simulink model "TPS_SWC"  (R2022b)
settings: configuration reference "TPS_AutosarConfig" (kept outside this file)
model workspace (MATLAB code in the model file):
  | cmdLim = Simulink.Parameter;
  | cmdLim.Value = 15;
  | cmdLim.Description = 'Limit for controlling the maximum surface command angle.';
  | cmdLim.Min = 0;
  | cmdLim.Max = 90;
  | cmdLim.DocUnits = 'deg';
  | 
  | dispGain = Simulink.Parameter;
  | dispGain.Value = 0.75;
  | dispGain.Description = 'Gain applied to the displacement error.';
  | dispGain.Min = 0;
  | dispGain.Max = [];
  | dispGain.DocUnits = 'deg/sec/deg';
  | 
  | dispLim = Simulink.Parameter;
  | dispLim.Value = 30;
  | dispLim.Description = 'Limit for controlling the maximum commanded angle.';
  | dispLim.Min = 0;
  | dispLim.Max = 180;
  | dispLim.DocUnits = 'deg';
  | 
  | intGain = Simulink.Parameter;
  | intGain.Value = 0.5;
  | intGain.Description = 'Gain applied to the integral error.';
  | intGain.Min = 0;
  | intGain.Max = [];
  | intGain.DocUnits = 'deg/sec/deg/sec';
  | 
  | intLim = Simulink.Parameter;
  | intLim.Value = 5;
  | intLim.Description = 'Limit for controlling the maximum commanded angle.';
  | intLim.Min = 0;
  | intLim.Max = 90;
  | intLim.DocUnits = 'deg';
  | 
  | rateGain = Simulink.Parameter;
  | rateGain.Value = 2;
  | rateGain.Description = 'Gain applied to the rate error.';
  | rateGain.Min = 0;
  | rateGain.Max = [];
  | rateGain.DocUnits = 'deg/deg/sec';
  | 
  | rateLim = Simulink.Parameter;
  | rateLim.Value = 6;
  | rateLim.Description = 'Limit for controlling the maximum commanded angle.';
  | rateLim.Min = 0;
  | rateLim.Max = 180;
  | rateLim.DocUnits = 'deg/sec';
  | 
  | hdgGain = Simulink.Parameter;
  | hdgGain.Value = 0.015;
values from neighbouring files (symbols this model uses):
  Dem_EventStatusType : value not decoded    [TPS_DD.sldd]
  TPS_SampleTime = 0.01    [TPS_DD.sldd]
libraries: autosarlibdem x4, autosarlibnvm x3, simulink x1
settings Model: RequirementInfo={} %GIDa_fe9045fd_0412_4b6e_8206_617cc20e6fde  DataDictionary=TPS_DD.sldd  FPTRunName=Active  Creator=MAAM  LastModifiedBy=MAAM
settings ConfigSetRef: SourceName=TPS_AutosarConfig

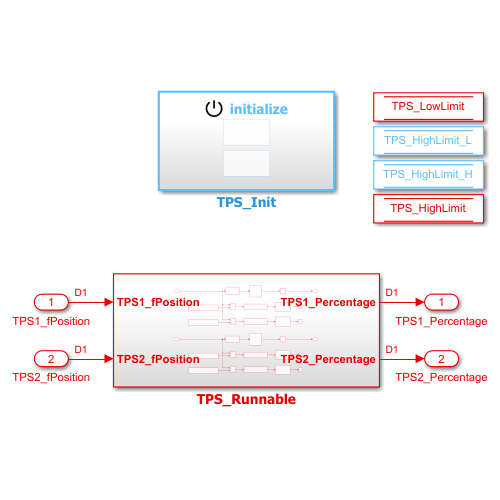
[thumbnail: Simulink's stored preview of the top-level diagram]
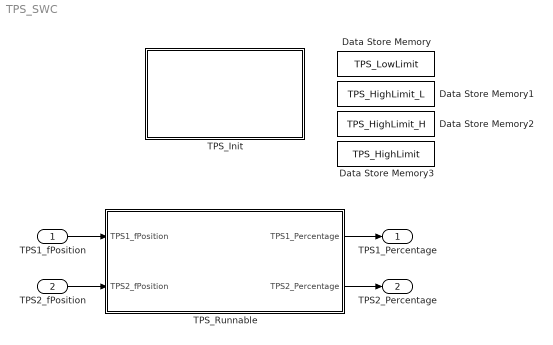
== system TPS_SWC ==
  TPS1_fPosition : Inport  OutDataTypeStr=uint16  SampleTime=TPS_SampleTime
  TPS2_fPosition : Inport  Port=2  OutDataTypeStr=uint16  SampleTime=TPS_SampleTime
  Data Store Memory : DataStoreMemory  DataStoreName=TPS_LowLimit  WriteAfterWriteMsg=warning  ShowAdditionalParam=off  OutDataTypeStr=uint8
  Data Store Memory1 : DataStoreMemory  DataStoreName=TPS_HighLimit_L  WriteAfterWriteMsg=warning  ShowAdditionalParam=off  OutDataTypeStr=uint8
  Data Store Memory2 : DataStoreMemory  DataStoreName=TPS_HighLimit_H  WriteAfterWriteMsg=warning  ShowAdditionalParam=off  OutDataTypeStr=uint8
  Data Store Memory3 : DataStoreMemory  DataStoreName=TPS_HighLimit  WriteAfterWriteMsg=warning  ShowAdditionalParam=off  OutDataTypeStr=uint16
  TPS_Init : Subsystem  TreatAsAtomicUnit=on
  TPS_Runnable : Subsystem  SystemSampleTime=1
  TPS1_Percentage : Outport  OutDataTypeStr=single  Unit=%
  TPS2_Percentage : Outport  Port=2  OutDataTypeStr=single  Unit=%
  wires:
  TPS1_fPosition/1 -> TPS_Runnable/1(TPS1_fPosition)
  TPS2_fPosition/1 -> TPS_Runnable/2(TPS2_fPosition)
  TPS_Runnable/1(TPS1_Percentage) -> TPS1_Percentage/1
  TPS_Runnable/2(TPS2_Percentage) -> TPS2_Percentage/1

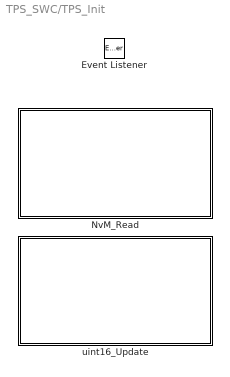
== system TPS_SWC/TPS_Init ==
  Event Listener : EventListener  DisableCoverage=on  EventName=reset
  NvM_Read : Subsystem  Tag=NvM_Read  Priority=1
  uint16_Update : Subsystem  Tag=uint16_Update  Priority=2

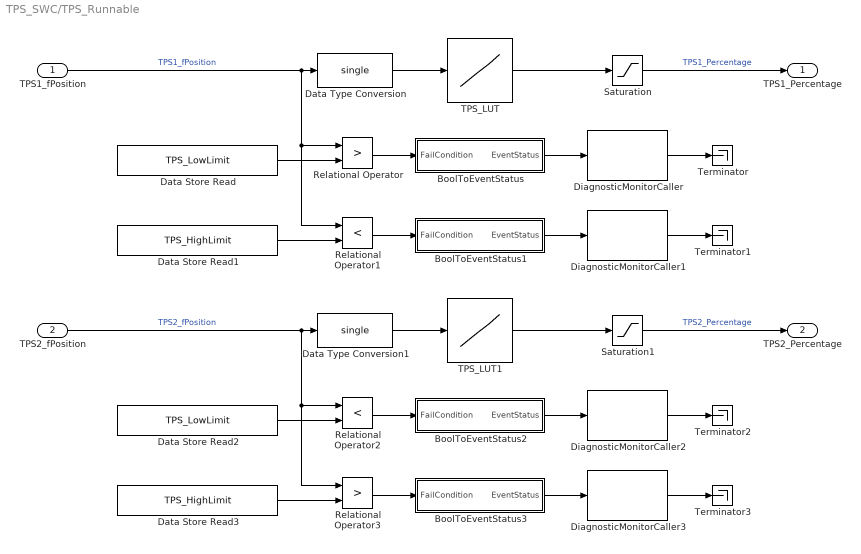
== system TPS_SWC/TPS_Runnable ==
  TPS1_fPosition : Inport  OutDataTypeStr=uint16
  TPS2_fPosition : Inport  Port=2  OutDataTypeStr=uint16
  BoolToEventStatus : Subsystem
  BoolToEventStatus1 : Subsystem
  BoolToEventStatus2 : Subsystem
  BoolToEventStatus3 : Subsystem
  Data Store Read : DataStoreRead  DataStoreName=TPS_LowLimit  IndexOptions=Index vector (dialog)  Indices=1  OutputSizes=1
  Data Store Read1 : DataStoreRead  DataStoreName=TPS_HighLimit  IndexOptions=Index vector (dialog)  Indices=1  OutputSizes=1
  Data Store Read2 : DataStoreRead  DataStoreName=TPS_LowLimit  IndexOptions=Index vector (dialog)  Indices=1  OutputSizes=1
  Data Store Read3 : DataStoreRead  DataStoreName=TPS_HighLimit  IndexOptions=Index vector (dialog)  Indices=1  OutputSizes=1
  Data Type Conversion : DataTypeConversion  OutDataTypeStr=single  SaturateOnIntegerOverflow=off  RndMeth=Floor
  Data Type Conversion1 : DataTypeConversion  OutDataTypeStr=single  SaturateOnIntegerOverflow=off  RndMeth=Floor
  DiagnosticMonitorCaller : autosarlibdem/DiagnosticMonitorCaller  PortName=TPS1_StuckLow  Operation=SetEventStatus  Datatype=Enum: Dem_EventStatusType  st=-1  ServiceImpl=autosar.bsw.DemDiagnosticMonitor
  DiagnosticMonitorCaller1 : autosarlibdem/DiagnosticMonitorCaller  PortName=TPS1_StuckHigh  Operation=SetEventStatus  Datatype=Enum: Dem_EventStatusType  st=-1  ServiceImpl=autosar.bsw.DemDiagnosticMonitor
  DiagnosticMonitorCaller2 : autosarlibdem/DiagnosticMonitorCaller  PortName=TPS2_StuckLow  Operation=SetEventStatus  Datatype=Enum: Dem_EventStatusType  st=-1  ServiceImpl=autosar.bsw.DemDiagnosticMonitor
  DiagnosticMonitorCaller3 : autosarlibdem/DiagnosticMonitorCaller  PortName=TPS2_StuckHigh  Operation=SetEventStatus  Datatype=Enum: Dem_EventStatusType  st=-1  ServiceImpl=autosar.bsw.DemDiagnosticMonitor
  Relational Operator : RelationalOperator  Operator=>  OutDataTypeStr=boolean  RndMeth=Simplest  InputSameDT=off
  Relational Operator1 : RelationalOperator  Operator=<  OutDataTypeStr=boolean  RndMeth=Simplest  InputSameDT=off
  Relational Operator2 : RelationalOperator  Operator=<  OutDataTypeStr=boolean  RndMeth=Simplest  InputSameDT=off
  Relational Operator3 : RelationalOperator  Operator=>  OutDataTypeStr=boolean  RndMeth=Simplest  InputSameDT=off
  Saturation : Saturate  UpperLimit=100  LowerLimit=0
  Saturation1 : Saturate  UpperLimit=100  LowerLimit=0
  TPS_LUT : Lookup_n-D  NumberOfTableDimensions=1  BreakpointsForDimension1=0:100:1000  BreakpointsForDimension1DataTypeStr=single  Table=0:10:100  TableDataTypeStr=single  InterpMethod=Nearest  ExtrapMethod=Clip  InternalRulePriority=Speed  OutDataTypeStr=single  RndMeth=Simplest
  TPS_LUT1 : Lookup_n-D  NumberOfTableDimensions=1  BreakpointsForDimension1=0:100:1000  BreakpointsForDimension1DataTypeStr=single  Table=0:10:100  TableDataTypeStr=single  InterpMethod=Nearest  InternalRulePriority=Speed  OutDataTypeStr=single  RndMeth=Simplest
  Terminator{,1..3} (4 alike) : Terminator
  TPS1_Percentage : Outport  OutDataTypeStr=single  Unit=%
  TPS2_Percentage : Outport  Port=2  OutDataTypeStr=single  Unit=%
  wires:
  Data Type Conversion1/1 -> TPS_LUT1/1
  TPS_LUT1/1 -> Saturation1/1
  Saturation1/1 -> TPS2_Percentage/1  "TPS2_Percentage"
  Data Store Read2/1 -> Relational Operator2/2
  Data Store Read3/1 -> Relational Operator3/2
  TPS2_fPosition/1 -> Relational Operator2/1, Relational Operator3/1, Data Type Conversion1/1  "TPS2_fPosition"
  Relational Operator2/1 -> BoolToEventStatus2/1(FailCondition)
  Relational Operator3/1 -> BoolToEventStatus3/1(FailCondition)
  BoolToEventStatus2/1(EventStatus) -> DiagnosticMonitorCaller2/1
  BoolToEventStatus3/1(EventStatus) -> DiagnosticMonitorCaller3/1
  BoolToEventStatus1/1(EventStatus) -> DiagnosticMonitorCaller1/1
  Relational Operator1/1 -> BoolToEventStatus1/1(FailCondition)
  Relational Operator/1 -> BoolToEventStatus/1(FailCondition)
  TPS1_fPosition/1 -> Data Type Conversion/1, Relational Operator1/1, Relational Operator/1  "TPS1_fPosition"
  Data Store Read1/1 -> Relational Operator1/2
  Data Store Read/1 -> Relational Operator/2
  Saturation/1 -> TPS1_Percentage/1  "TPS1_Percentage"
  TPS_LUT/1 -> Saturation/1
  Data Type Conversion/1 -> TPS_LUT/1
  BoolToEventStatus/1(EventStatus) -> DiagnosticMonitorCaller/1
  DiagnosticMonitorCaller/1 -> Terminator/1
  DiagnosticMonitorCaller1/1 -> Terminator1/1
  DiagnosticMonitorCaller2/1 -> Terminator2/1
  DiagnosticMonitorCaller3/1 -> Terminator3/1

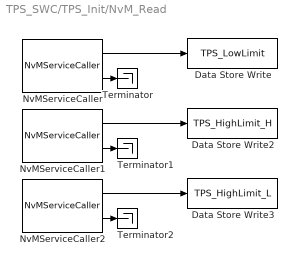
== system TPS_SWC/TPS_Init/NvM_Read ==
  Data Store Write : DataStoreWrite  DataStoreName=TPS_LowLimit  IndexOptions=Index vector (dialog)  Indices=1  OutputSizes=1
  Data Store Write2 : DataStoreWrite  DataStoreName=TPS_HighLimit_H  IndexOptions=Index vector (dialog)  Indices=1  OutputSizes=1
  Data Store Write3 : DataStoreWrite  DataStoreName=TPS_HighLimit_L  IndexOptions=Index vector (dialog)  Indices=1  OutputSizes=1
  NvMServiceCaller : autosarlibnvm/NvMServiceCaller  PortName=TPS_LowLimit_NvMService  Operation=ReadBlock  ArgumentSpecification=TPS_LowLimit_ID  st=-1  ServiceImpl=autosar.bsw.NvMService
  NvMServiceCaller1 : autosarlibnvm/NvMServiceCaller  PortName=TPS_HighLimit_H_NvMService  Operation=ReadBlock  ArgumentSpecification=TPS_HighLimit_ID_H  st=-1  ServiceImpl=autosar.bsw.NvMService
  NvMServiceCaller2 : autosarlibnvm/NvMServiceCaller  PortName=TPS_HighLimit_L_NvMService  Operation=ReadBlock  ArgumentSpecification=TPS_HighLimit_ID_L  st=-1  ServiceImpl=autosar.bsw.NvMService
  Terminator : Terminator
  Terminator1 : Terminator
  Terminator2 : Terminator
  wires:
  NvMServiceCaller1/1 -> Data Store Write2/1
  NvMServiceCaller/2 -> Terminator/1
  NvMServiceCaller2/2 -> Terminator2/1
  NvMServiceCaller/1 -> Data Store Write/1
  NvMServiceCaller1/2 -> Terminator1/1
  NvMServiceCaller2/1 -> Data Store Write3/1

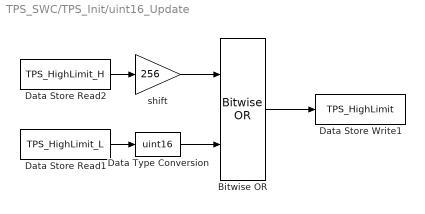
== system TPS_SWC/TPS_Init/uint16_Update ==
  Bitwise OR : simulink/Logic and Bit Operations/Bitwise Operator  logicop=OR  UseBitMask=off  NumInputPorts=2  BitMask=bin2dec('11011001')  BitMaskRealWorld=Stored Integer
      settings: LibrarySourceBlock=|
      | simulink/Quick Insert/Logic and Bit
      | Operations/Bitwise OR
  Data Store Read1 : DataStoreRead  DataStoreName=TPS_HighLimit_L  IndexOptions=Index vector (dialog)  Indices=1  OutputSizes=1
  Data Store Read2 : DataStoreRead  DataStoreName=TPS_HighLimit_H  IndexOptions=Index vector (dialog)  Indices=1  OutputSizes=1
  Data Store Write1 : DataStoreWrite  DataStoreName=TPS_HighLimit  IndexOptions=Index vector (dialog)  Indices=1  OutputSizes=1
  Data Type Conversion : DataTypeConversion  OutDataTypeStr=uint16  SaturateOnIntegerOverflow=off  RndMeth=Floor
  shift : Gain  Gain=256  OutDataTypeStr=uint16
  wires:
  Bitwise OR/1 -> Data Store Write1/1
  Data Store Read1/1 -> Data Type Conversion/1
  shift/1 -> Bitwise OR/1
  Data Type Conversion/1 -> Bitwise OR/2
  Data Store Read2/1 -> shift/1

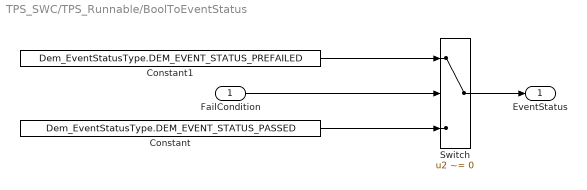
== system TPS_SWC/TPS_Runnable/BoolToEventStatus ==
  FailCondition : Inport
  Constant : Constant  Value=Dem_EventStatusType.DEM_EVENT_STATUS_PASSED
  Constant1 : Constant  Value=Dem_EventStatusType.DEM_EVENT_STATUS_PREFAILED
  Switch : Switch  Criteria=u2 ~= 0  SaturateOnIntegerOverflow=off  InputSameDT=off
  EventStatus : Outport  VectorParamsAs1DForOutWhenUnconnected=off
  wires:
  FailCondition/1 -> Switch/2
  Constant/1 -> Switch/3
  Constant1/1 -> Switch/1
  Switch/1 -> EventStatus/1

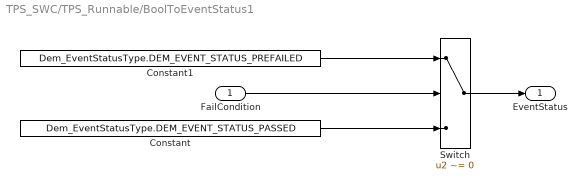
== system TPS_SWC/TPS_Runnable/BoolToEventStatus1 ==
  FailCondition : Inport
  Constant : Constant  Value=Dem_EventStatusType.DEM_EVENT_STATUS_PASSED
  Constant1 : Constant  Value=Dem_EventStatusType.DEM_EVENT_STATUS_PREFAILED
  Switch : Switch  Criteria=u2 ~= 0  SaturateOnIntegerOverflow=off  InputSameDT=off
  EventStatus : Outport  VectorParamsAs1DForOutWhenUnconnected=off
  wires:
  Switch/1 -> EventStatus/1
  Constant1/1 -> Switch/1
  Constant/1 -> Switch/3
  FailCondition/1 -> Switch/2

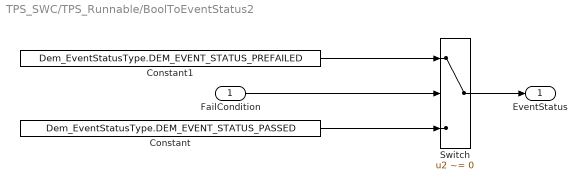
== system TPS_SWC/TPS_Runnable/BoolToEventStatus2 ==
  FailCondition : Inport
  Constant : Constant  Value=Dem_EventStatusType.DEM_EVENT_STATUS_PASSED
  Constant1 : Constant  Value=Dem_EventStatusType.DEM_EVENT_STATUS_PREFAILED
  Switch : Switch  Criteria=u2 ~= 0  SaturateOnIntegerOverflow=off  InputSameDT=off
  EventStatus : Outport  VectorParamsAs1DForOutWhenUnconnected=off
  wires:
  Switch/1 -> EventStatus/1
  Constant1/1 -> Switch/1
  Constant/1 -> Switch/3
  FailCondition/1 -> Switch/2

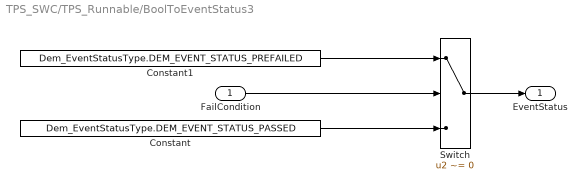
== system TPS_SWC/TPS_Runnable/BoolToEventStatus3 ==
  FailCondition : Inport
  Constant : Constant  Value=Dem_EventStatusType.DEM_EVENT_STATUS_PASSED
  Constant1 : Constant  Value=Dem_EventStatusType.DEM_EVENT_STATUS_PREFAILED
  Switch : Switch  Criteria=u2 ~= 0  SaturateOnIntegerOverflow=off  InputSameDT=off
  EventStatus : Outport  VectorParamsAs1DForOutWhenUnconnected=off
  wires:
  FailCondition/1 -> Switch/2
  Constant/1 -> Switch/3
  Constant1/1 -> Switch/1
  Switch/1 -> EventStatus/1
